simulink model "bai2"  (R2017b)
settings: Solver=ode5  StartTime=0.0  StopTime=800  FixedStep=0.1  RelTol=1e-3
libraries: fuzblock x1
settings Model: Creator=phamt  LastModifiedBy=phamt

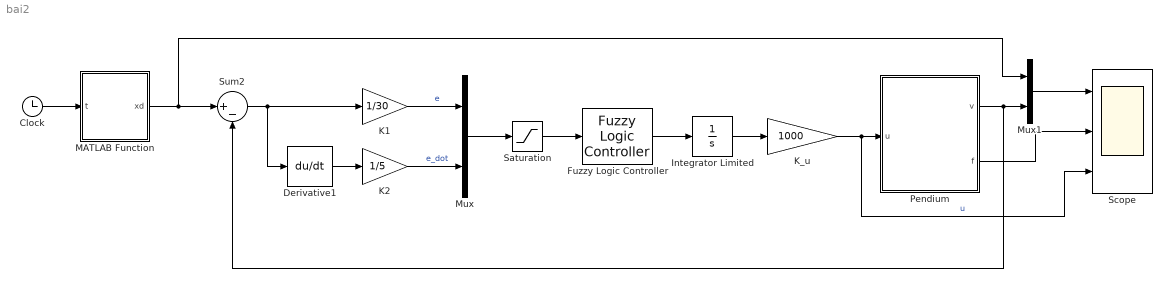
== system bai2 ==
  Clock : Clock
      settings: Decimation=800
  Derivative1 : Derivative
  Fuzzy Logic Controller : fuzblock/Fuzzy Logic  Controller  FIS='bai1_PD_FIS.fis'  OutputSampleNumber=101  DataType=double  FuzzifiedInputs=off  RuleFiringStrengths=off  RuleOutputs=off  AggregatedOutputs=off  SimulateUsing=Interpreted execution
  Integrator Limited : Integrator  LimitOutput=on  UpperSaturationLimit=1  LowerSaturationLimit=-1
  K1 : Gain  Gain=1/30
  K2 : Gain  Gain=1/5
  K_u : Gain  Gain=1000
  MATLAB Function : MATLAB Function  TreatAsAtomicUnit=on
  Mux : Mux  Inputs=2
  Mux1 : Mux  Inputs=2
  Pendium : Subsystem  mask{m=1300, Ap=0.3, d=100, t=0.2, v0=0, f0=0}
  Saturation : Saturate  UpperLimit=1  LowerLimit=-1
  Scope : Scope  NumInputPorts=3
  Sum2 : Sum  Inputs=|+-
  wires:
  MATLAB Function/1(xd) -> Mux1/1, Sum2/1
  Derivative1/1 -> K2/1
  Clock/1 -> MATLAB Function/1(t)
  Mux/1 -> Saturation/1
  K2/1 -> Mux/2  "e_dot"
  Sum2/1 -> Derivative1/1, K1/1
  Fuzzy Logic Controller/1 -> Integrator Limited/1
  K1/1 -> Mux/1  "e"
  Saturation/1 -> Fuzzy Logic Controller/1
  Mux1/1 -> Scope/1
  Integrator Limited/1 -> K_u/1
  Pendium/1(v) -> Sum2/2, Mux1/2
  K_u/1 -> Scope/3, Pendium/1(u)  "u"
  Pendium/2(f) -> Scope/2

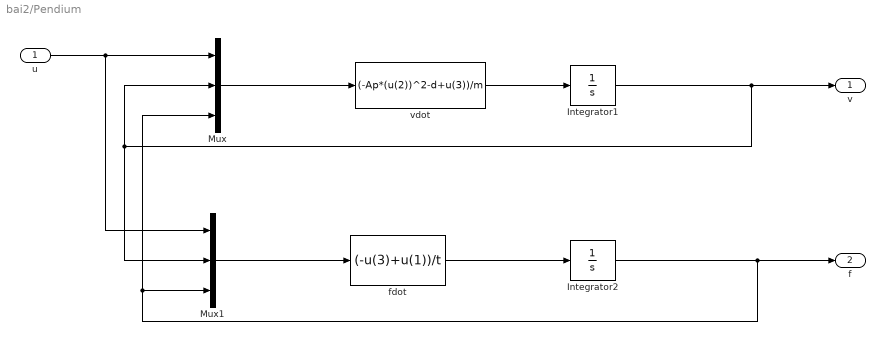
== system bai2/Pendium ==
  u : Inport
  Integrator1 : Integrator  InitialCondition=v0
  Integrator2 : Integrator  InitialCondition=f0
  Mux : Mux  Inputs=3
  Mux1 : Mux  Inputs=3
  fdot : Fcn  Expr=(-u(3)+u(1))/t
  vdot : Fcn  Expr=(-Ap*(u(2))^2-d+u(3))/m
  v : Outport
  f : Outport  Port=2
  wires:
  Integrator2/1 -> Mux1/3, Mux/3, f/1
  Integrator1/1 -> Mux1/2, Mux/2, v/1
  vdot/1 -> Integrator1/1
  fdot/1 -> Integrator2/1
  u/1 -> Mux1/1, Mux/1
  Mux1/1 -> fdot/1
  Mux/1 -> vdot/1

== matlab function bai2/MATLAB Function ==
  data: t input; xd output
function xd = fcn(t)
if (0<=t) && (t<100)  
    xd = 30;
elseif (100<=t) &&(t<200) 
    xd = 20;
elseif (200<=t) &&(t<400)  
    xd = 10;
elseif (400<=t) &&(t<500)  
    xd = 25;
elseif (500<=t) &&(t<600)  
    xd = 15;
elseif (600<=t) &&(t<800)  
    xd = 30;
else xd = 0;
end
end
